simulink model "GalvoModel_v31_CC"  (R2013a)
settings: Solver=ode45  StartTime=0.0  StopTime=50e-3  RelTol=1e-3
PreLoadFcn:
  | Kp_cc=evalin('base',paramCtrl.Kp_cc);
InitFcn:
  | Kp_cc=evalin('base',paramCtrl.Kp_cc);
libraries: simulink x1
settings Model: BufferReuse=off  Creator=mainster  LastModifiedBy=mainster
settings DataIOCC: SaveOutput=off  SaveTime=off
settings OptimizationCC: InlineParams=on  BufferReuse=off
settings DebuggingCC: InitInArrayFormatMsg=none
settings ModelReferenceCC: ModelReferenceNumInstancesAllowed=Single

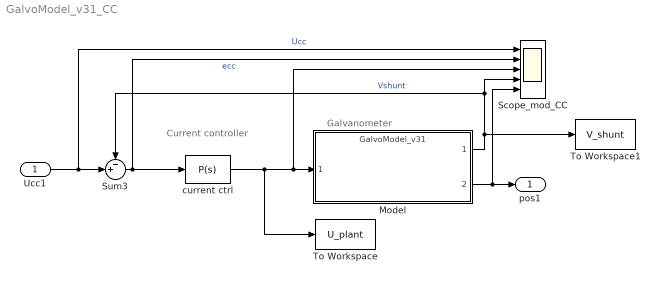
== system GalvoModel_v31_CC ==
  note: Current controller
  note: Galvanometer
  Ucc1 : Inport
  Model : ModelReference  ModelNameDialog=GalvoModel_v31.slx  SimulationMode=Normal  ModelReferenceVersion=1.15  CopyOfModelName=GalvoModel_v31.slx  DefaultDataLogging=on
      mask Display:
      | str=sprintf('%s',get(gcbh,'ModelName'));
      | port_label('input', 1, 'VCoil','texmode','on')
      | color('blue');
      | port_label('output', 1, 'VShunt','texmode','on')
      | color('black');
      | port_label('output', 2, 'AngPos')
      | %text(.05,.98,['{\fontsize{12}\it\bf' strrep(str,'_',' ') '}'],'horizontalAlignment','left','verticalAlignment','top','texmode','on')
      | text(.05,.98,['{\fontsize{12}\it\bf' strrep(str,'_','\_') '}'],'horizontalAlignment','left','verticalAlignment','top','texmode','on')
      | 
      | %get_param(gcbh,'Location')
      | % pos = get_param(gcb, 'Position');
      | % width = pos(3) - pos(1);
      | % x = [0, width];
      | % y = ones(1,length(x))*0.8;
      | % plot(x,y)
  Scope_mod_CC : Scope  NumInputPorts=5
      settings: ShowLegends=on  TimeRange=0.03  YMin=-1~-1~-1~-0.02~0  YMax=3~3~3~0.06~0.02  MaxDataPoints=500000
  Sum3 : Sum  Inputs=-+|
  To Workspace : ToWorkspace  VariableName=U_plant  SampleTime=-1  SaveFormat=Timeseries
  To Workspace1 : ToWorkspace  VariableName=V_shunt  SampleTime=-1  SaveFormat=Timeseries
  current ctrl : simulink/Continuous/PID Controller  Controller=P  TimeDomain=Continuous-time  SampleTime=1  IntegratorMethod=Forward Euler  FilterMethod=Forward Euler  Form=Parallel  P=Kp_cc  I=0.7525  D=0.156  N=100  InitialConditionSource=internal  InitialConditionForIntegrator=0  InitialConditionForFilter=0  ExternalReset=none  LimitOutput=off  UpperSaturationLimit=25  LowerSaturationLimit=-25  LinearizeAsGain=off  AntiWindupMode=none  Kb=1  TrackingMode=off  Kt=1  PParamMin=[]  PParamMax=[]  IParamMin=[]  IParamMax=[]  DParamMin=[]  DParamMax=[]  NParamMin=[]  NParamMax=[]  KbParamMin=[]  KbParamMax=[]  KtParamMin=[]  KtParamMax=[]  POutMin=[]  POutMax=[]  IOutMin=[]  IOutMax=[]  DOutMin=[]  DOutMax=[]  NOutMin=[]  NOutMax=[]  KbOutMin=[]  KbOutMax=[]  KtOutMin=[]  KtOutMax=[]  IntegratorOutMin=[]  IntegratorOutMax=[]  FilterOutMin=[]  FilterOutMax=[]  SumOutMin=[]  SumOutMax=[]  SumI1OutMin=[]  SumI1OutMax=[]  SumI2OutMin=[]  SumI2OutMax=[]  SumI3OutMin=[]  SumI3OutMax=[]  SumDOutMin=[]  SumDOutMax=[]  SaturationOutMin=[]  SaturationOutMax=[]  IntegratorContinuousStateAttributes=''  IntegratorStateMustResolveToSignalObject=off  IntegratorRTWStateStorageClass=Auto  FilterContinuousStateAttributes=''  FilterStateMustResolveToSignalObject=off  FilterRTWStateStorageClass=Auto
  pos1 : Outport
  wires:
  Model/2 -> Scope_mod_CC/5, pos1/1
  Ucc1/1 -> Scope_mod_CC/1, Sum3/2  "Ucc"
  Sum3/1 -> Scope_mod_CC/2, current ctrl/1  "ecc"
  current ctrl/1 -> To Workspace/1, Scope_mod_CC/3, Model/1
  Model/1 -> Scope_mod_CC/4, Sum3/1, To Workspace1/1  "Vshunt"
